simulink model "FM_Transmitter_Basics_2"  (R2022a)
settings: Solver=FixedStepDiscrete  StartTime=0.0  StopTime=inf  RelTol=1e-3
libraries: commsynccomp2 x1, dspvision x1, dspsigops x1, matrix_library x1
settings Model: Creator=vovan  LastModifiedBy=vovan

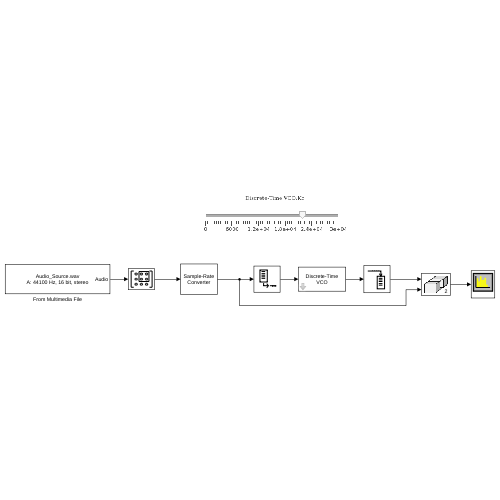
[thumbnail: Simulink's stored preview of the top-level diagram]
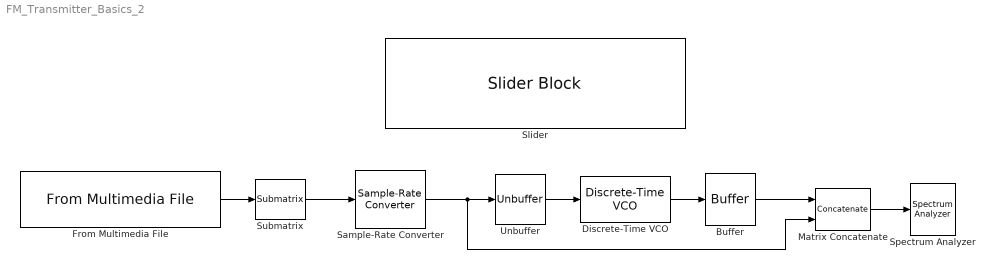
== system FM_Transmitter_Basics_2 ==
  Buffer : Buffer  N=1000  OutputFrames=off
  Discrete-Time VCO : commsynccomp2/Discrete-Time VCO  Ac=1  Fc=100e3  Kc=21798.42967375118  Ph=0  ts=-1
      settings: SourceProductBaseCode=CM
  From Multimedia File : dspvision/From Multimedia File  inputFilename=wav/Audio_Source.wav  readRange=[1 Inf]  loop=on  numPlays=inf  outputStreams=Audio only  videoDataType=single  audioDataType=double  inheritSampleTime=on  userDefinedSampleTime=1/30  noAudioOutput=off  isIntensityVideo=off  fourcc=RGB  colorVideoFormat=Separate color signals  outputEOF=off  dataOrg=Column-major  audioFrameSize=100  computeAudioFrameSize=off  outSamplingMode=Sample based
  Matrix Concatenate : Concatenate  Mode=Multidimensional array  ConcatenateDimension=2
  Sample-Rate Converter : dspsigops/Sample-Rate Converter  InputSampleRate=44100  OutputSampleRate=10*44100  OutputRateTolerance=0  Bandwidth=40e3  StopbandAttenuation=80  SimulateUsing=Code generation
      settings: SourceProductBaseCode=DS
  Slider : SliderBlock  ScaleMax=30e3
  Spectrum Analyzer : SpectrumAnalyzer
  Submatrix : matrix_library/Submatrix  RowSpan=All rows  RowStartMode=First  RowStartIndex=1  RowEndMode=Last  RowEndIndex=1  ColSpan=Range of columns  ColStartMode=First  ColStartIndex=1  ColEndMode=Index  ColEndIndex=1
      settings: SourceProductBaseCode=SL
  Unbuffer : Unbuffer
  wires:
  From Multimedia File/1 -> Submatrix/1
  Sample-Rate Converter/1 -> Unbuffer/1, Matrix Concatenate/2
  Discrete-Time VCO/1 -> Buffer/1
  Submatrix/1 -> Sample-Rate Converter/1
  Matrix Concatenate/1 -> Spectrum Analyzer/1
  Unbuffer/1 -> Discrete-Time VCO/1
  Buffer/1 -> Matrix Concatenate/1
